simulink model "Derivative_System"  (R2024a)
settings: Solver=FixedStepDiscrete  StartTime=0.0  StopTime=10.0  FixedStep=0.01  RelTol=1e-3
values from neighbouring files (symbols this model uses):
  Ts = 0.01    [Derivative_System_try_1.sldd]
settings Model: DataDictionary=Derivative_System_try_1.sldd  Creator=ntyler  LastModifiedBy=ntyler

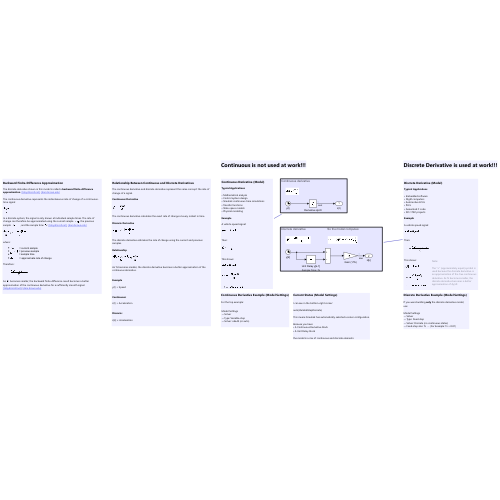
[thumbnail: Simulink's stored preview of the top-level diagram]
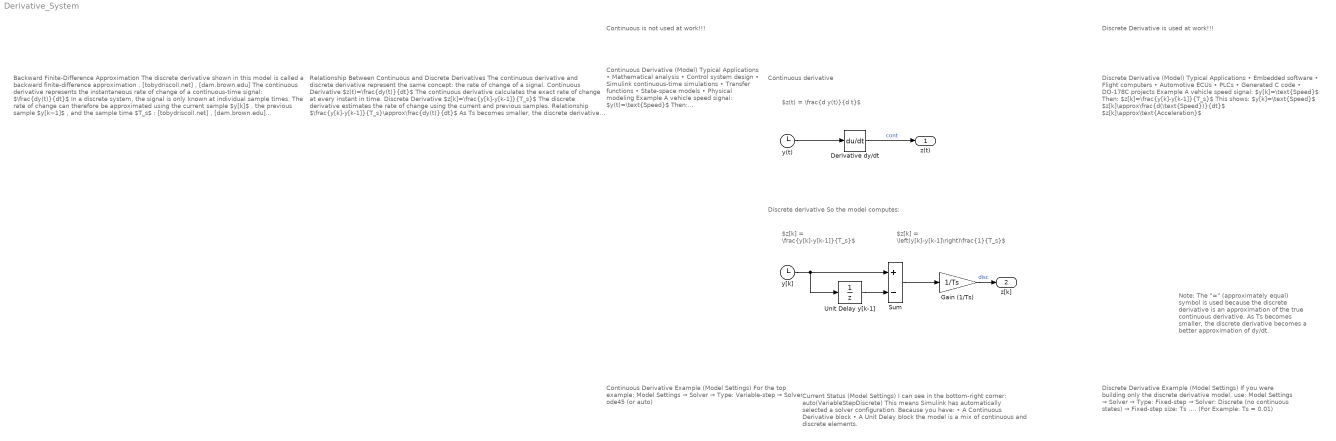
== system Derivative_System ==
  note: Backward Finite-Difference Approximation
      | The discrete derivative shown in this model is called a backward finite-difference approximation . [tobydriscoll.net] , [dam.brown.edu]
      | The continuous derivative represents the instantaneous rate of change of a continuous-time signal:
      | $\frac{dy(t)}{dt}$
      | In a discrete system, the signal is only known at individual sample times. The rate of change can therefore be approximated using the current sample $y[k]$ , the previous sample $y[k−1]$ , and the sample time $T_s$ : [tobydriscoll.net] , [dam.brown.edu]
      | $\frac{dy(t)}{dt}\approx\frac{y[k]-y[k-1]}{T_s}$
      | where:
      | $y[k]$ = current sample
      | $y[k−1]$ = previous sample
      | $T_s$ ​ = sample time
      | $z[k]$ = approximate rate of change
      | Therefore:
      | $z[k]=\frac{y[k]-y[k-1]}{T_s}$
      | As $T_s$ ​ becomes smaller, the backward finite-difference result becomes a better approximation of the continuous derivative for a sufficiently smooth signal. [tobydriscoll.net] , [dam.brown.edu]
      |
      | ​
  note: Discrete Derivative Example (Model Settings)
      |
      | If you were building only the discrete derivative model, use:
      |
      | Model Settings
      | → Solver
      | → Type: Fixed-step
      | → Solver: Discrete (no continuous states)
      | → Fixed-step size: Ts .... (For Example: Ts = 0.01)
      | ​
      |
      | ​
      |
      | ​
  note: Continuous Derivative Example (Model Settings)
      | For the top example:
      |
      | Model Settings
      | → Solver
      | → Type: Variable-step
      | → Solver: ode45 (or auto)
      |
      | ​
  note: Relationship Between Continuous and Discrete Derivatives
      |
      | The continuous derivative and discrete derivative represent the same concept: the rate of change of a signal.
      |
      | Continuous Derivative
      |
      | $z(t)=\frac{dy(t)}{dt}$
      |
      | The continuous derivative calculates the exact rate of change at every instant in time.
      |
      | Discrete Derivative
      |
      | $z[k]=\frac{y[k]-y[k-1]}{T_s}$
      |
      | The discrete derivative estimates the rate of change using the current and previous samples.
      |
      | Relationship
      |
      | $\frac{y[k]-y[k-1]}{T_s}\approx\frac{dy(t)}{dt}$
      |
      | As Ts becomes smaller, the discrete derivative becomes a better approximation of the continuous derivative.
      |
      | Example
      |
      | y(t) = Speed
      |
      | Continuous:
      |
      | z(t) = Acceleration
      |
      | Discrete:
      |
      | z[k] ≈ Acceleration
      |
      | ​
  note: Current Status (Model Settings)
      |
      | I can see in the bottom-right corner:
      |
      | auto(VariableStepDiscrete)
      |
      | This means Simulink has automatically selected a solver configuration.
      |
      | Because you have:
      | • A Continuous Derivative block
      | • A Unit Delay block
      |
      | the model is a mix of continuous and discrete elements.
  note: Note:
      |
      | The "≈" (approximately equal) symbol is used because the discrete derivative is an approximation of the true continuous derivative. As Ts becomes smaller, the discrete derivative becomes a better approximation of dy/dt.
  note: Continuous Derivative (Model)
      | Typical Applications
      | • Mathematical analysis
      | • Control system design
      | • Simulink continuous-time simulations
      | • Transfer functions
      | • State-space models
      | • Physical modeling
      | Example
      | A vehicle speed signal:
      | $y(t)=\text{Speed}$
      |
      | Then:
      | $z(t)=\frac{dy(t)}{dt}$
      |
      | This shows:
      | $y(t)=\text{Speed}$
      |
      | $z(t)=\frac{d(\text{Speed})}{dt}$
      |
      | $z(t)=\text{Acceleration}$
      |
      | ​
      |
      | ​
      |
      | ​
      |
      | ​
  note: Continuous derivative
  note: $z(t) = \frac{d y(t)}{d t}$
  note: Discrete derivative So the model computes:
  note: $z[k] = \frac{y[k]-y[k-1]}{T_s}$
  note: $z[k] = \left(y[k]-y[k-1]\right)\frac{1}{T_s}$
  note: Discrete Derivative (Model)
      | Typical Applications
      | • Embedded software
      | • Flight computers
      | • Automotive ECUs
      | • PLCs
      | • Generated C code
      | • DO-178C projects
      | Example
      | A vehicle speed signal:
      | $y[k]=\text{Speed}$
      |
      | Then:
      | $z[k]=\frac{y[k]-y[k-1]}{T_s}$
      |
      | This shows:
      | $y[k]=\text{Speed}$
      |
      | $z[k]\approx\frac{d(\text{Speed})}{dt}$
      | $z[k]\approx\text{Acceleration}$
      |
      | ​
  note: Continuous is not used at work!!!
  note: Discrete Derivative is used at work!!!
  Derivative dy/dt : Derivative
  Gain (1/Ts) : Gain  Gain=1/Ts
  Sum : Sum  Inputs=+-
  Unit Delay y[k-1] : UnitDelay  SampleTime=Ts  HasFrameUpgradeWarning=on
      settings: AttributesFormatString=Sample Time: %<SampleTime>
  y(t) : Clock
  y[k] : Clock
  z(t) : Outport
  z[k] : Outport  Port=2
  wires:
  y(t)/1 -> Derivative dy/dt/1
  Derivative dy/dt/1 -> z(t)/1  "cont"
  y[k]/1 -> Sum/1, Unit Delay y[k-1]/1
  Sum/1 -> Gain (1/Ts)/1
  Unit Delay y[k-1]/1 -> Sum/2
  Gain (1/Ts)/1 -> z[k]/1  "disc"
